simulink model "MRACROBOTG12"  (R2025a)
settings: Solver=VariableStepAuto  StartTime=0.0  StopTime=10.0  RelTol=1e-3
InitFcn:
  | % --- INICIO DEL CÓDIGO InitFcn ---
  | 
  | % 1. (¡CAMBIA ESTO!) Asegúrate de que esta ruta sea correcta
  | addpath('C:/RoboDK/Matlab/');
  | 
  | % 2. Declarar las variables como globales para que Simulink las vea
  | global RDK;
  | global ROBOT;
  | 
  | % 3. Iniciar la conexión con RoboDK
  | RDK = Robolink();
  | 
  | % 4. (¡CAMBIA ESTO!) Pon el nombre exacto de tu robot en RoboDK
  | robot_name = 'Fanuc CRX-5iA';
  | ROBOT = RDK.Item(robot_name, RDK.ITEM_TYPE_ROBOT);
  | 
  | % 5. Comprobar que se encontró
  | if ~ROBOT.Valid()
  |     % Si el script falla aquí, es porque no encontró tu robot.
  |     error('No se encontró el robot: %s', robot_name);
  | end
  | 
  | % 6. Configurar el modo para simulación en tiempo real
  | RDK.setRunMode(RDK.RUNMODE_SIMULATE);
  | 
  | % 7. Mensaje de éxito
  | fprintf('¡RoboDK y el robot "%s" conectados a Simulink!\n', robot_name);
  | 
  | % --- FIN DEL CÓDIGO ---
libraries: robotmaniplib x1, robotsim3dlib x1, sim3dlib x1
settings Model: Creator=Sandro  LastModifiedBy=jaros

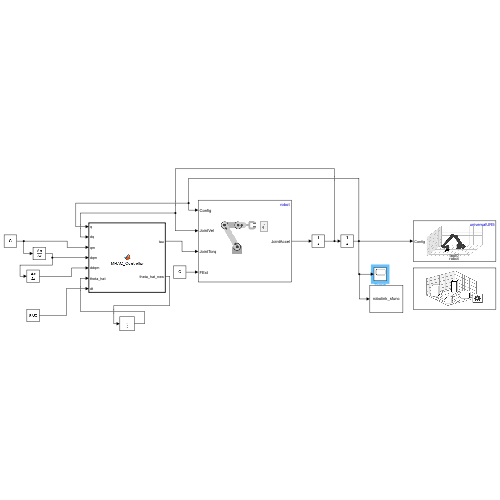
[thumbnail: Simulink's stored preview of the top-level diagram]
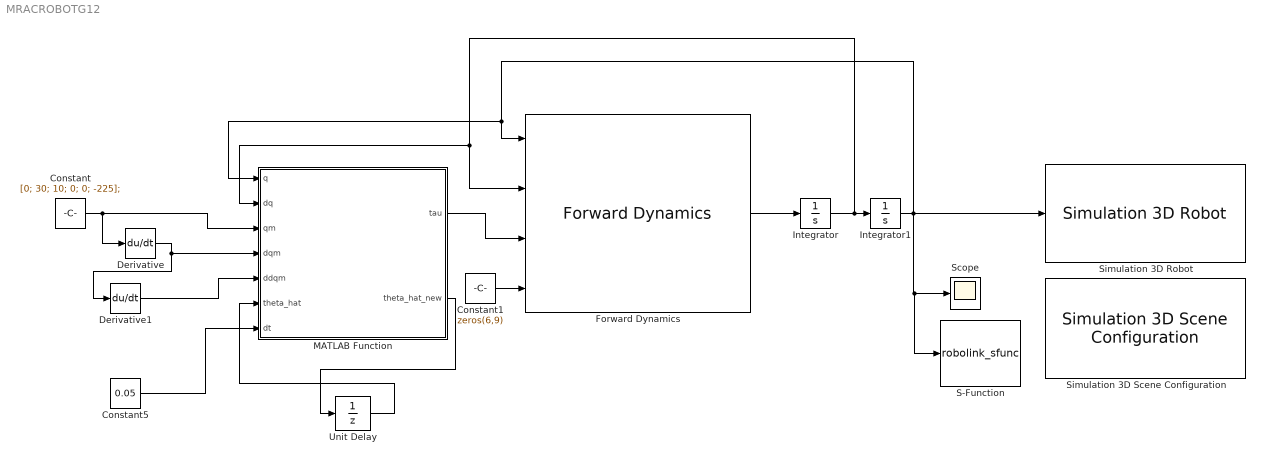
== system MRACROBOTG12 ==
  Constant : Constant  Value=[0; 30; 10; 0; 0; -225];
  Constant1 : Constant  Value=zeros(6,9)
  Constant5 : Constant  Value=0.05
  Derivative : Derivative
  Derivative1 : Derivative
  Forward Dynamics : robotmaniplib/Forward Dynamics  RigidBodyTree=robot  SimulateUsing=Interpreted execution
  Integrator : Integrator
  Integrator1 : Integrator
  MATLAB Function : MATLAB Function  TreatAsAtomicUnit=on
  S-Function : S-Function  FunctionName=robolink_sfunc  SFunctionDeploymentMode=off  EnableBusSupport=off
  Scope : Scope
      settings: ActiveDisplayYMinimum=-3.5259077169502433  ActiveDisplayYMaximum=2.1192008294047175
  Simulation 3D Robot : robotsim3dlib/Simulation 3D Robot  actorInputType=Robot Library  RigidBodyTree=universalUR5  ActorName=robot  existActorChekBox=off  initialTrans=[0 0 0]  initialRot=[0 0 0]  initialConfig="[0  0  0  0  0  0]"  EndEffector=tool0  eeOffsetInpChekBox=off  eeTargetTrans=[0 0 0]  eeTargetRot=[0 0 0]  enableRegionGraspChekBox=off  regionGraspInpChekBox=off  eeTargTransDiff=[0.2 0.2 0.2]  eeTargRotDiff=[0 0 0]  enableVisualVisualization=on  enableCollisionVisualization=off  collisionGeomColor=[0 1 0]  collisionGeomTransp=0.1  inpConfEnbVal=on  inpGraspEnbVal=off  inpTransEnbVal=off  outConfEnbVal=off  outGraspEnbVal=off  outTransEnbVal=off  SampleTime=0.01  ActorType=SimulinkVehicle  ID=C  aMode=6  ActorTag=robot  Mesh=RigidBodyTree
  Simulation 3D Scene Configuration : sim3dlib/Simulation 3D Scene Configuration  Priority=0  ProjectFormat=Default Scenes  SceneDesc=Curved road  ProjectName=C:\Program Files\MATLAB\R2025a\toolbox\shared\sim3d_projects\automotive_project_windows\UE\WindowsNoEditor\VehicleSimulation.exe  ScenePath=/Game/Maps/EmptyScene  EnableOpenDRIVE=off  vehTagList={'<empty>';'Custom';'Scene Origin';'robot'}  vehTag=Scene Origin  AttachedCameraRelativeTranslation=[0 0 0]  FreeCameraDefaultInitialTranslation=[-6, 0, 2]  AttachedCameraRelativeRotation=[0 0 0]  FreeCameraDefaultInitialRotation=[0, -15, 0]  ViewpointName=Custom  FreeCameraInitialTranslation=[0 0 0]  ViewpointTranslation=[0 0 0]  FreeCameraInitialRotation=[0 0 0]  ViewpointRotation=[0 0 0]  OpVisEn=off  Ts=0.02  EnableWindow=on  EnableRemoteAccess=off  EnableWeather=off  SunAzimuth=90  SunAltitude=40.0  EnableGeospatialSun=off  Latitude=0  Longitude=0  Date=2023-01-01  Time=10:30:00  GeoTimeZone=-5.0  SunDaylightSaving=off  wind=1  clouds=10  EnableVolumetricClouds=off  CloudCoverage=0  CloudAltitude=6  fog=0  rain=0  RaindropsEffect=off  SnowDensity=0  EnableGeospatial=off  TilesetSource=Earth terrain  UseTrueOrigin=off  OriginHeight=200  OriginLatitude=40.744652  OriginLongitude=-73.988864  MapStyle=Aerial  AdditionalAssetIDs=[]  UseAdvancedSunSky=off  SolarTime=11  TimeZone=-5  Day=21  Month=9  Year=2022  UseDaylightSavingTime=on  DSTStartDay=10  DSTStartMonth=3  DSTEndDay=3  DSTEndMonth=11  DSTSwitchHour=2  sensorTag=MainCamera1  sensorId=1  sensorName=MainCamera1  mountLoc=Origin  offsetFlag=off  tmountOffset=[0, 0, 0]  rmountOffset=[0, 0, 0]  HorizontalResolution=1280  VerticalResolution=720  HorizontalFOV=60  mountPoint=[0 0 0]  mountOrientation=[0 0 0]  aMode=6  ID=1  GeoTrigger=Inactive  ViewNameList={'Custom'}  ViewTranslationList={'[0 0 0]'}  ViewRotationList={'[0 0 0]'}
      settings: LibrarySourceBlock=robotsim3dlib/Simulation 3D Scene Configuration
  Unit Delay : UnitDelay  InitialCondition=zeros(12,1)  SampleTime=-1  HasFrameUpgradeWarning=on
  wires:
  Forward Dynamics/1 -> Integrator/1
  Integrator/1 -> Forward Dynamics/2, MATLAB Function/2(dq), Integrator1/1
  Integrator1/1 -> Simulation 3D Robot/1, S-Function/1, Scope/1, Forward Dynamics/1, MATLAB Function/1(q)
  Constant1/1 -> Forward Dynamics/4
  Constant/1 -> Derivative/1, MATLAB Function/3(qm)
  MATLAB Function/1(tau) -> Forward Dynamics/3
  MATLAB Function/2(theta_hat_new) -> Unit Delay/1
  Unit Delay/1 -> MATLAB Function/6(theta_hat)
  Constant5/1 -> MATLAB Function/7(dt)
  Derivative/1 -> Derivative1/1, MATLAB Function/4(dqm)
  Derivative1/1 -> MATLAB Function/5(ddqm)

== matlab function MRACROBOTG12/MATLAB Function ==
  data: q input; dq input; tau output; qm input; dqm input; ddqm input; theta_hat input; dt input; theta_hat_new output
function [tau, theta_hat_new] = MRAC_Controller(q, dq, qm, dqm, ddqm, theta_hat, dt)
%#codegen
% Controlador Adaptativo MRAC para robot manipulador de 6 ejes (Fanuc CRX-5iA)
%
% Entradas:
%   q         -> posición actual [6x1]
%   dq        -> velocidad actual [6x1]
%   qm        -> posición deseada [6x1]
%   dqm       -> velocidad deseada [6x1]
%   ddqm      -> aceleración deseada [6x1]
%   theta_hat -> estimación actual de parámetros [12x1]
%   dt        -> paso de integración (ej. 0.001)
%
% Salidas:
%   tau           -> torque de control [6x1]
%   theta_hat_new -> parámetros actualizados [12x1]

%% === Parámetros de control ===
Kp     = 15 * eye(6);   % Ganancia proporcional
Kd     = 10 * eye(6);   % Ganancia derivativa
Gamma  = 5  * eye(12);  % Matriz de adaptación

%% === Cálculo de errores ===
e  = qm - q;     % error de posición
de = dqm - dq;   % error de velocidad

%% === Señal de error filtrado ===
r = de + 2*e;    % filtro simple para estabilidad (λ=2)

%% === Matriz de regresión Y (simplificada para el MRAC) ===
% Dimensiones: Y [6x12]
% Cada fila representa los términos asociados a un eje del robot
% (en una implementación real, incluiría dinámicas del modelo)
Y = zeros(6,12);
for i = 1:6
    Y(i,:) = [ddqm(i), dqm(i), qm(i), de(i), e(i), 1, ...
              dq(i), q(i), sin(q(i)), cos(q(i)), dqm(i)*e(i), e(i)^2];
end

%% === Ley de control MRAC ===
% τ = Y*θ̂ + Kd*de + Kp*e
tau = Y * theta_hat + Kd * de + Kp * e;

%% === Ley adaptativa ===
% 𝜃̇̂ = -Γ * Yᵗ * r
theta_hat_dot = -Gamma * (Y') * r;

%% === Integración de parámetros ===
theta_hat_new = theta_hat + dt * theta_hat_dot;

end
